simulink model "modele_simulink"  (R2022b)
settings: Solver=VariableStepAuto  StartTime=0.0  StopTime=140  RelTol=1e-3
values from neighbouring files (symbols this model uses):
  A = [0,1,0 ... (first row only)    [script_matlab.m]
  amax = 2.3    [script_matlab.m]
  B = [0;0;1/tau]    [script_matlab.m]
  h = 0.6    [script_matlab.m]
  kd = 0.7    [script_matlab.m]
  kp = 0.2    [script_matlab.m]
  L = 3    [script_matlab.m]
  ns = 3    [script_matlab.m]
  r = 2.5    [script_matlab.m]
  tmax = 12    [script_matlab.m]
  z1 = [0;0;0]    [script_matlab.m]
settings Model: Creator=bouquet18u  LastModifiedBy=antoi
settings ModelReferenceCC: EnableRefExpFcnMdlSchedulingChecks=on

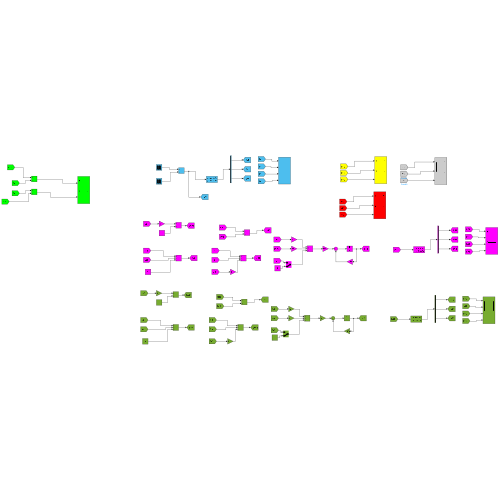
[thumbnail: Simulink's stored preview of the top-level diagram]
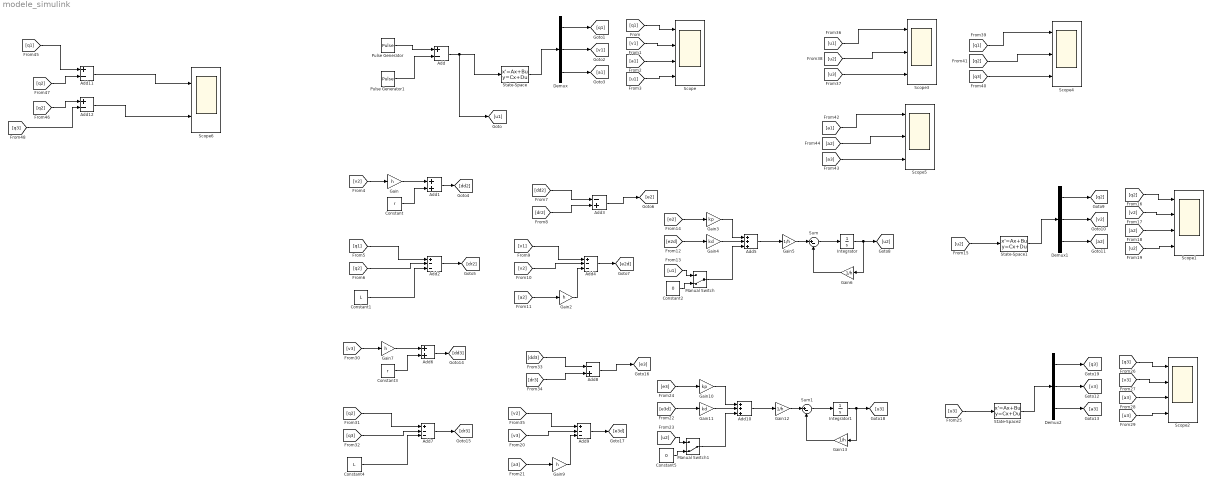
== system modele_simulink ==
  Add : Sum  Inputs=+-
  Add1 : Sum
  Add10 : Sum  Inputs=+++
  Add11 : Sum  Inputs=+-
  Add12 : Sum  Inputs=+-
  Add{2,4,7,9} (4 alike) : Sum  Inputs=+--
  Add3 : Sum  Inputs=-+
  Add5 : Sum  Inputs=+++
  Add6 : Sum
  Add8 : Sum  Inputs=-+
  Constant : Constant  Value=r
  Constant1 : Constant  Value=L
  Constant2 : Constant  Value=0
  Constant3 : Constant  Value=r
  Constant4 : Constant  Value=L
  Constant5 : Constant  Value=0
  Demux : Demux  Outputs=3
  Demux1 : Demux  Outputs=3
  Demux2 : Demux  Outputs=3
  Gain{,2,7,9} (4 alike) : Gain  Gain=h
  Gain10 : Gain  Gain=kp
  Gain11 : Gain  Gain=kd
  Gain{5..6,12..13} (4 alike) : Gain  Gain=1/h
  Gain3 : Gain  Gain=kp
  Gain4 : Gain  Gain=kd
  Integrator : Integrator
  Integrator1 : Integrator
  Manual Switch : ManualSwitch  CurrentSetting=0
  Manual Switch1 : ManualSwitch  CurrentSetting=0
  Pulse Generator : DiscretePulseGenerator  PulseType=Time based  Amplitude=amax  Period=4*tmax  PulseWidth=50
  Pulse Generator1 : DiscretePulseGenerator  PulseType=Time based  Amplitude=amax  Period=4*tmax  PulseWidth=50  PhaseDelay=tmax
  Scope : Scope  NumInputPorts=4
  Scope1 : Scope  NumInputPorts=4
  Scope2 : Scope  NumInputPorts=4
  Scope3 : Scope  NumInputPorts=3
  Scope4 : Scope  NumInputPorts=3
  Scope5 : Scope  NumInputPorts=3
  Scope6 : Scope  NumInputPorts=2
  State-Space : StateSpace  A=A  B=B  C=eye(ns)  D=zeros(ns,1)  InitialCondition=z1  ParameterTunability=Unconstrained
  State-Space1 : StateSpace  A=A  B=B  C=eye(ns)  D=zeros(ns,1)  InitialCondition=z1  ParameterTunability=Unconstrained
  State-Space2 : StateSpace  A=A  B=B  C=eye(ns)  D=zeros(ns,1)  InitialCondition=z1  ParameterTunability=Unconstrained
  Sum : Sum  Inputs=|+-
  Sum1 : Sum  Inputs=|+-
  wires:
  Pulse Generator/1 -> Add/1
  Pulse Generator1/1 -> Add/2
  State-Space/1 -> Demux/1
  Add/1 -> [u1], State-Space/1
  Demux/1 -> [q1]
  Demux/2 -> [v1]
  Demux/3 -> [a1]
  [q1] -> Scope/1
  [v1] -> Scope/2
  [a1] -> Scope/3
  [u1] -> Scope/4
  [v2] -> Gain/1
  Gain/1 -> Add1/1
  Constant/1 -> Add1/2
  Add1/1 -> [dd2]
  Add2/1 -> [dr2]
  [q2] -> Add2/2
  Constant1/1 -> Add2/3
  [dd2] -> Add3/1
  [dr2] -> Add3/2
  Add3/1 -> [e2]
  [a2] -> Gain2/1
  [v1] -> Add4/1
  [v2] -> Add4/2
  Gain2/1 -> Add4/3
  Add4/1 -> [e2d]
  [e2] -> Gain3/1
  Gain3/1 -> Add5/1
  [e2d] -> Gain4/1
  Gain4/1 -> Add5/2
  Constant2/1 -> Manual Switch/2
  [u1] -> Manual Switch/1
  Manual Switch/1 -> Add5/3
  Add5/1 -> Gain5/1
  Gain5/1 -> Sum/1
  Sum/1 -> Integrator/1
  Integrator/1 -> Gain6/1, [u2]
  Gain6/1 -> Sum/2
  [u2] -> Scope1/4
  Demux1/1 -> [q2]
  [q2] -> Scope1/1
  State-Space1/1 -> Demux1/1
  [v2] -> Scope1/2
  [a2] -> Scope1/3
  Demux1/3 -> [a2]
  Demux1/2 -> [v2]
  [u2] -> State-Space1/1
  Constant5/1 -> Manual Switch1/2
  Manual Switch1/1 -> Add10/3
  Add10/1 -> Gain12/1
  [u2] -> Manual Switch1/1
  Demux2/3 -> [a3]
  [v3] -> Scope2/2
  Demux2/1 -> [q3]
  [u3] -> Scope2/4
  State-Space2/1 -> Demux2/1
  [q3] -> Scope2/1
  Gain12/1 -> Sum1/1
  Integrator1/1 -> Gain13/1, [u3]
  Sum1/1 -> Integrator1/1
  Demux2/2 -> [v3]
  Gain13/1 -> Sum1/2
  [e3d] -> Gain11/1
  [a3] -> Scope2/3
  Gain10/1 -> Add10/1
  Constant4/1 -> Add7/3
  [a3] -> Gain9/1
  Constant3/1 -> Add6/2
  Gain9/1 -> Add9/3
  [dr3] -> Add8/2
  [v2] -> Add9/1
  [v3] -> Gain7/1
  [u3] -> State-Space2/1
  Add7/1 -> [dr3]
  [e3] -> Gain10/1
  [q3] -> Add7/2
  [v3] -> Add9/2
  [dd3] -> Add8/1
  Add8/1 -> [e3]
  Gain11/1 -> Add10/2
  Gain7/1 -> Add6/1
  Add6/1 -> [dd3]
  Add9/1 -> [e3d]
  [u1] -> Scope3/1
  [u2] -> Scope3/2
  [u3] -> Scope3/3
  [q3] -> Scope4/3
  [q1] -> Scope4/1
  [q2] -> Scope4/2
  [a2] -> Scope5/2
  [a1] -> Scope5/1
  [a3] -> Scope5/3
  [q1] -> Add2/1
  [q2] -> Add7/1
  [q1] -> Add11/1
  [q2] -> Add11/2
  [q2] -> Add12/1
  [q3] -> Add12/2
  Add11/1 -> Scope6/1
  Add12/1 -> Scope6/2
